simulink model "model8"  (Simulink 7.7)
settings: Solver=ode45  StartTime=0.0  StopTime=10  RelTol=1e-3
values from neighbouring files (symbols this model uses):
  tstep = 0.1    [lab8.m]
libraries: simulink x2
settings Model: Creator=student  LastModifiedBy=mestan
settings DataIOCC: LimitDataPoints=off

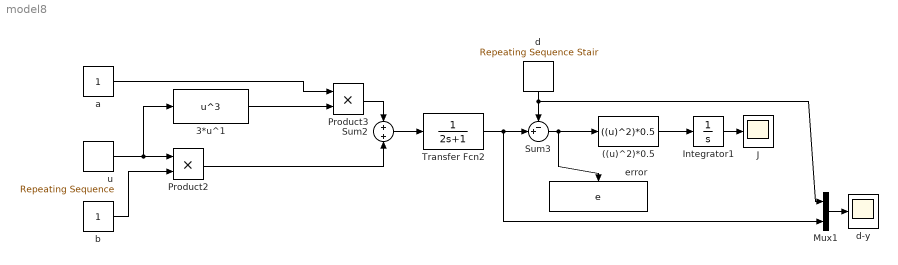
== system model8 ==
  ((u)^2)*0.5 : Fcn  Expr=((u)^2)*0.5
  3*u^1 : MATLABFcn  MATLABFcn=u^3
  Integrator1 : Integrator
  J : Scope
      settings: SaveName=ScopeData3
  Mux1 : Mux  Inputs=2
  Product2 : Product  RndMeth=Zero
  Product3 : Product  RndMeth=Zero
  Sum2 : Sum  Inputs=+|+
  Sum3 : Sum  Inputs=-+|
  Transfer Fcn2 : TransferFcn  Denominator=[2 1]
  a : Constant
  b : Constant
  d : simulink/Sources/Repeating Sequence Stair  SystemSampleTime=-1  OutValues=d  tsamp=tstep  OutMin=[]  OutMax=[]  OutDataTypeStr=double  OutputDataTypeScalingMode=double  OutDataType=fixdt(0,8)  ConRadixGroup=Best Precision: Vector-wise  OutScaling=2^-12
  d-y : Scope
      settings: SaveName=ScopeData2
  error : ToWorkspace  VariableName=e  SampleTime=tstep  SaveFormat=Array
  u : simulink/Sources/Repeating Sequence  SystemSampleTime=-1  rep_seq_t=t  rep_seq_y=u
      link override Look-Up Table1: Table=rep_seq_y  RndMeth=Round
  wires:
  3*u^1/1 -> Product3/2
  Sum2/1 -> Transfer Fcn2/1
  Product3/1 -> Sum2/1
  Product2/1 -> Sum2/2
  Transfer Fcn2/1 -> Sum3/2, Mux1/2
  Sum3/1 -> error/1, ((u)^2)*0.5/1
  a/1 -> Product3/1
  d/1 -> Sum3/1, Mux1/1
  u/1 -> Product2/1, 3*u^1/1
  b/1 -> Product2/2
  ((u)^2)*0.5/1 -> Integrator1/1
  Mux1/1 -> d-y/1
  Integrator1/1 -> J/1
